simulink model "cccvlgorithmfinall"  (R2018b)
settings: Solver=VariableStepAuto  StartTime=0.0  StopTime=400  RelTol=1e-3
undefined symbols (not defined in the file): Ion, Lithium
libraries: powerlib x24, simulink x4, electricdrivelib x1, powerlib_meascontrol x1
settings Model: Creator=PARTO  LastModifiedBy=PARTO

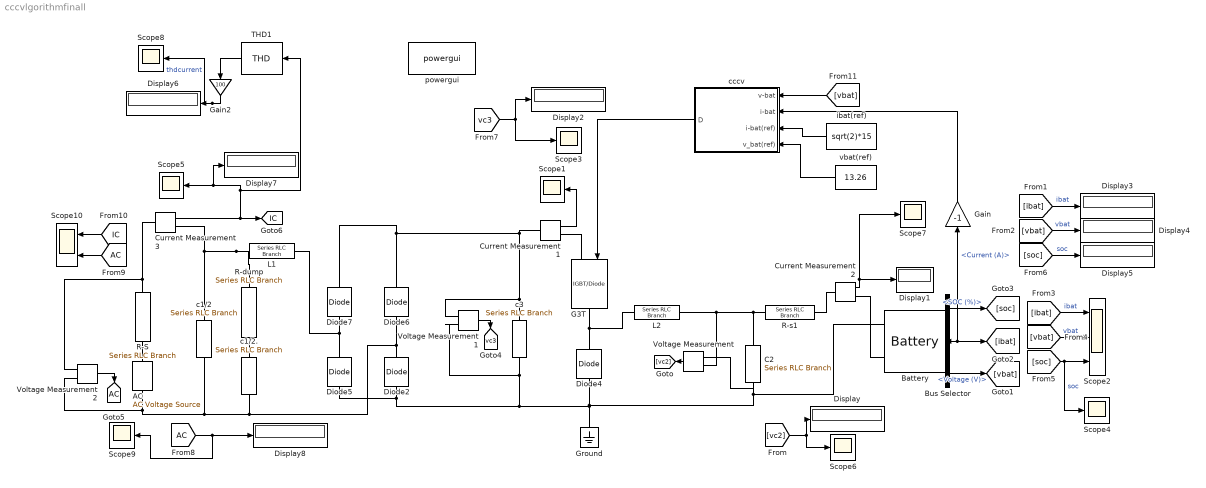
== system cccvlgorithmfinall ==
  AC : powerlib/Electrical Sources/AC Voltage Source  Amplitude=sqrt(2)*220  Phase=0  Frequency=50  SampleTime=0  Measurements=Voltage  BusType=PV  Pref=3.3e3  Qref=0  Qmin=-inf  Qmax=+inf
      settings: SourceProductName=Simscape Electrical
  Battery : electricdrivelib/Extra Sources/Battery  BatType=Lithium-Ion  ShowTempParam=off  ThermalPreset=no  ShowAgeParam=off  NomV=11.4  NomQ=5.4  SOC=19  Batt_Tr=30  PresetModel=on  MaxQ=5.4  MinV=8.55  FullV=13.2695  Dis_rate=2.3478  R=0.021111  Normal_OP=4.8835  expZone="[12.3164     0.265304]"  current=[6.5 13 32.5]  Units=Time  Tci=20  NomT=20  T2=-30  MaxQ2=4.8  FullV2=7.1  Normal_OP2=5.655  expZone2="[6.58           1]"  Rca=0.6  ti=2000  Dp=0  Neq0=0  Tsim=1e6  Ta1=25  Qeol=5.4*0.9  Reol=0.013333*1.2  Char_age=[2.3478, 3]  Dis_age=[2.3478, 10]  N1=1500  N2=10500  N3=1000  N4=1400  Ta2=45  N5=950
      settings: SourceProductName=Simscape Electrical
  Bus Selector : BusSelector  OutputSignals=SOC (%),Current (A),Voltage (V)
  C2 : powerlib/Elements/Series RLC Branch  LConnTagsString=__new0  RConnTagsString=__new0  BranchType=C  Resistance=1  Inductance=1e-3  SetiL0=off  InitialCurrent=0  Capacitance=700e-6  Setx0=off  InitialVoltage=0  Measurements=None
      settings: SourceProductName=Simscape Electrical
  Current Measurement1 : powerlib/Measurements/Current Measurement  PhasorSimulation=off  OutputType=Complex  PSBequivalent=0
      settings: SourceProductName=Simscape Electrical
  Current Measurement2 : powerlib/Measurements/Current Measurement  PhasorSimulation=off  OutputType=Complex  PSBequivalent=0
      settings: SourceProductName=Simscape Electrical
  Current Measurement3 : powerlib/Measurements/Current Measurement  PhasorSimulation=off  OutputType=Complex  PSBequivalent=0
      settings: SourceProductName=Simscape Electrical
  Diode{2,5..7} (4 alike) : powerlib/Power Electronics/Diode  Ron=0.000002  Lon=0.000002  Vf=0.8  IC=0  UseSnubber=0  Rs=0  Cs=0  Measurements=off
      settings: SourceProductName=Simscape Electrical
  Diode4 : powerlib/Power Electronics/Diode  Ron=0  Lon=0  Vf=0.8  IC=0  UseSnubber=0  Rs=0  Cs=0  Measurements=off
      settings: SourceProductName=Simscape Electrical
  Display{,1..8} (9 alike) : Display
  G3T : powerlib/Power Electronics/IGBT//Diode  Ron=1e-3  Rs=1e5  Cs=inf  Measurements=off
      settings: SourceProductName=Simscape Electrical
  Gain : Gain  Gain=-1
  Gain2 : Gain  Gain=100
  Ground : powerlib/Elements/Ground  LConnTagsString=a
      settings: SourceProductName=Simscape Electrical
  L1 : powerlib/Elements/Series RLC Branch  LConnTagsString=__new0  RConnTagsString=__new0  BranchType=L  Resistance=1  Inductance=5e-3  SetiL0=off  InitialCurrent=0  Capacitance=1e-6  Setx0=off  InitialVoltage=0  Measurements=None
      settings: SourceProductName=Simscape Electrical
  L2 : powerlib/Elements/Series RLC Branch  LConnTagsString=__new0  RConnTagsString=__new0  BranchType=L  Resistance=1  Inductance=1.5e-3  SetiL0=off  InitialCurrent=0  Capacitance=1e-6  Setx0=off  InitialVoltage=0  Measurements=None
      settings: SourceProductName=Simscape Electrical
  R-S : powerlib/Elements/Series RLC Branch  LConnTagsString=__new0  RConnTagsString=__new0  BranchType=R  Resistance=1e-6  Inductance=1e-3  SetiL0=off  InitialCurrent=0  Capacitance=1e-6  Setx0=off  InitialVoltage=0  Measurements=None
      settings: SourceProductName=Simscape Electrical
  "R-dump " : powerlib/Elements/Series RLC Branch  LConnTagsString=__new0  RConnTagsString=__new0  BranchType=R  Resistance=128  Inductance=1e-3  SetiL0=off  InitialCurrent=0  Capacitance=1e-6  Setx0=off  InitialVoltage=0  Measurements=None
      settings: SourceProductName=Simscape Electrical
  R-s1 : powerlib/Elements/Series RLC Branch  LConnTagsString=__new0  RConnTagsString=__new0  BranchType=R  Resistance=0.005  Inductance=1e-3  SetiL0=off  InitialCurrent=0  Capacitance=1e-6  Setx0=off  InitialVoltage=0  Measurements=None
      settings: SourceProductName=Simscape Electrical
  Scope{1,3..9} (8 alike) : Scope
  Scope10 : Scope  NumInputPorts=2
  Scope2 : Scope  NumInputPorts=3
  THD1 : powerlib_meascontrol/Measurements/THD  Freq=50  Ts=0
      settings: SourceProductName=Simscape Electrical
  Voltage Measurement : powerlib/Measurements/Voltage Measurement  PhasorSimulation=off  OutputType=Complex  PSBequivalent=0
      settings: SourceProductName=Simscape Electrical
  Voltage Measurement1 : powerlib/Measurements/Voltage Measurement  PhasorSimulation=off  OutputType=Complex  PSBequivalent=0
      settings: SourceProductName=Simscape Electrical
  Voltage Measurement2 : powerlib/Measurements/Voltage Measurement  PhasorSimulation=off  OutputType=Complex  PSBequivalent=0
      settings: SourceProductName=Simscape Electrical
  c1/2 : powerlib/Elements/Series RLC Branch  LConnTagsString=__new0  RConnTagsString=__new0  BranchType=C  Resistance=1  Inductance=1e-3  SetiL0=off  InitialCurrent=0  Capacitance=250e-6  Setx0=off  InitialVoltage=0  Measurements=None
      settings: SourceProductName=Simscape Electrical
  c1/2. : powerlib/Elements/Series RLC Branch  LConnTagsString=__new0  RConnTagsString=__new0  BranchType=C  Resistance=1  Inductance=1e-3  SetiL0=off  InitialCurrent=0  Capacitance=250e-6  Setx0=off  InitialVoltage=0  Measurements=None
      settings: SourceProductName=Simscape Electrical
  c3 : powerlib/Elements/Series RLC Branch  LConnTagsString=__new0  RConnTagsString=__new0  BranchType=C  Resistance=1  Inductance=1e-3  SetiL0=off  InitialCurrent=0  Capacitance=1000e-6  Setx0=off  InitialVoltage=0  Measurements=None
      settings: SourceProductName=Simscape Electrical
  cccv : Subsystem
  ibat(ref) : Constant  Value=sqrt(2)*15
  powergui : powerlib/powergui  Priority=1  SimulationMode=Continuous  SampleTime=50e-6  frequency=60  Iterations=50  frequencyindice=0  Pbase=100e6  ErrMax=1e-4  UnitsV=kV  UnitsW=MW  buscounter=0  FunctionMessages=off  echomessages=off  EnableUseOfTLC=off  CurrentSourceSwitches=off  DisableSnubberDevices=off  DisableRonSwitches=off  DisableVfSwitches=off  DisplayEquations=off  SolverType=Tustin/Backward Euler (TBE)  Interpol=off  ExternalGateDelay=off  methode=off  Ts=100  x0status=blocks  SPID=on  SwTol=0  HookPort=off  RestoreLinks=warning  ResistiveCurrentMeasurement=off  Frange=[0:2:500]  Ylog=off  Xlog=on  ShowGrid=off  save=off  variable=ZData  structure=0  ZoomFFT=off  StartTime=0.0  cycles=1  DisplayStyle=1  fundamental=60  FreqAxis=off  MaxFrequency=1000  frequencyindicesteady=1  RmsSteady=1  display=off
  vbat(ref) : Constant  Value=13.26
  tag scope: AC=global, IC=global, vc3=global
  wires:
  Current Measurement2/1 -> Scope7/1, Display1/1
  Bus Selector/2 -> [ibat], Gain/1  "<Current (A)>"
  Battery/1 -> Bus Selector/1
  Current Measurement1/1 -> Scope1/1
  Voltage Measurement/1 -> [vc2]
  [vc2] -> Scope6/1, Display/1
  [ibat] -> Scope2/1  "ibat"
  Bus Selector/1 -> [soc]  "<SOC (%)>"
  [soc] -> Scope4/1, Scope2/3  "soc"
  [vbat] -> Scope2/2  "vbat"
  Bus Selector/3 -> [vbat]  "<Voltage (V)>"
  [ibat] -> Display3/1  "ibat"
  [vbat] -> Display4/1  "vbat"
  [soc] -> Display5/1  "soc"
  THD1/1 -> Gain2/1
  Gain2/1 -> Scope8/1, Display6/1  "thdcurrent"
  Current Measurement3/1 -> [IC], THD1/1, Display7/1, Scope5/1
  Voltage Measurement1/1 -> [vc3]
  [vc3] -> Display2/1, Scope3/1
  Voltage Measurement2/1 -> [AC]
  [AC] -> Scope9/1, Display8/1
  [IC] -> Scope10/1
  [AC] -> Scope10/2
  Gain/1 -> cccv/2(i-bat)
  [vbat] -> cccv/1(v-bat)
  cccv/1(D) -> G3T/1
  ibat(ref)/1 -> cccv/3(i-bat(ref))
  vbat(ref)/1 -> cccv/4(v_bat(ref))
  connections:
  Battery/LConn2 -- Ground/LConn1 -- c3/RConn1 -- Voltage Measurement1/LConn2 -- Diode2/LConn1 -- Diode5/LConn1 -- Diode4/LConn1 -- Voltage Measurement/LConn2 -- C2/RConn1
  G3T/RConn1 -- Diode4/RConn1 -- L2/LConn1
  c3/LConn1 -- Voltage Measurement1/LConn1 -- Diode6/RConn1 -- Diode7/RConn1 -- Current Measurement1/LConn1
  L1/LConn1 -- "R-dump "/LConn1 -- c1/2/LConn1 -- Current Measurement3/RConn1
  Diode6/LConn1 -- Diode2/RConn1 -- c1/2./RConn1 -- Voltage Measurement2/LConn2 -- AC/LConn1 -- c1/2/RConn1
  Diode5/RConn1 -- L1/RConn1 -- Diode7/LConn1
  R-s1/LConn1 -- L2/RConn1 -- Voltage Measurement/LConn1 -- C2/LConn1
  R-s1/RConn1 -- Current Measurement2/LConn1
  Current Measurement1/RConn1 -- G3T/LConn1
  Current Measurement2/RConn1 -- Battery/LConn1
  "R-dump "/RConn1 -- c1/2./LConn1
  Current Measurement3/LConn1 -- Voltage Measurement2/LConn1 -- R-S/RConn1
  AC/RConn1 -- R-S/LConn1

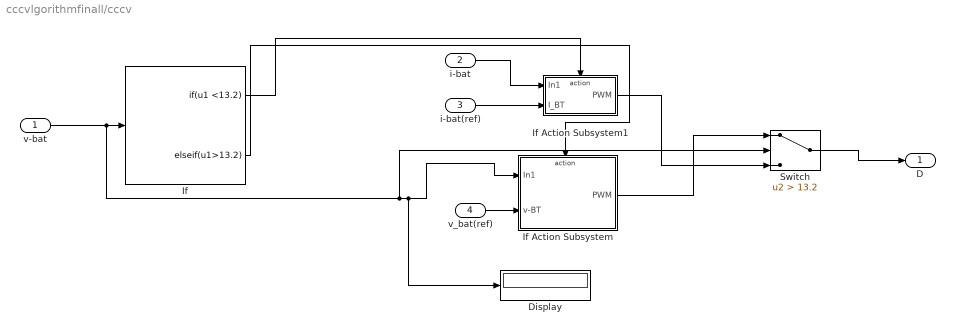
== system cccvlgorithmfinall/cccv ==
  v-bat : Inport
  i-bat : Inport  Port=2
  i-bat(ref) : Inport  Port=3
  v_bat(ref) : Inport  Port=4
  Display : Display
  If : If  IfExpression=u1 <13.2  ElseIfExpressions=u1>13.2  ShowElse=off
  If Action Subsystem : Subsystem  TreatAsAtomicUnit=on
  If Action Subsystem1 : Subsystem  TreatAsAtomicUnit=on
  Switch : Switch  Criteria=u2 > Threshold  Threshold=13.2
  D : Outport
  wires:
  If/1 -> If Action Subsystem1/Action
  i-bat/1 -> If Action Subsystem1/1(In1)
  If/2 -> If Action Subsystem/Action
  i-bat(ref)/1 -> If Action Subsystem1/2(I_BT)
  v_bat(ref)/1 -> If Action Subsystem/2(v-BT)
  v-bat/1 -> Switch/2, Display/1, If Action Subsystem/1(In1), If/1
  If Action Subsystem/1(PWM) -> Switch/1
  If Action Subsystem1/1(PWM) -> Switch/3
  Switch/1 -> D/1

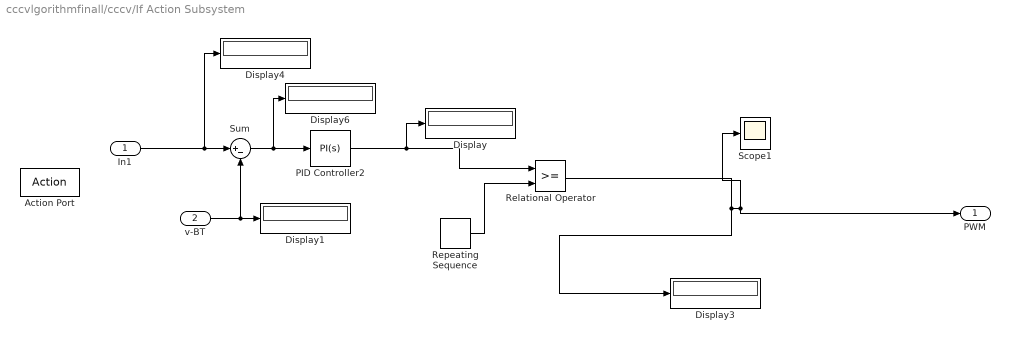
== system cccvlgorithmfinall/cccv/If Action Subsystem ==
  In1 : Inport
  v-BT : Inport  Port=2
  Action Port : ActionPort  ActionType=elseif
  Display{,1,3..4,6} (5 alike) : Display
  PID Controller2 : simulink/Continuous/PID Controller  Controller=PI  Form=Parallel  TimeDomain=Continuous-time  SampleTime=-1  IntegratorMethod=Forward Euler  FilterMethod=Forward Euler  ControllerParametersSource=internal  P=100  I=1  D=0  UseFilter=on  N=100  TunerSelectOption=Transfer Function Based (PID Tuner App)  InitialConditionSource=internal  InitialConditionForIntegrator=0  InitialConditionForFilter=0  DifferentiatorICPrevScaledInput=0  ExternalReset=none  TrackingMode=off  Kt=1  LimitOutput=off  UpperSaturationLimit=inf  LowerSaturationLimit=-inf  LinearizeAsGain=on  AntiWindupMode=none  Kb=1  POutMin=[]  POutMax=[]  IOutMin=[]  IOutMax=[]  DOutMin=[]  DOutMax=[]  NOutMin=[]  NOutMax=[]  SumOutMin=[]  SumOutMax=[]  SaturationOutMin=[]  SaturationOutMax=[]  PParamMin=[]  PParamMax=[]  IParamMin=[]  IParamMax=[]  DParamMin=[]  DParamMax=[]  NParamMin=[]  NParamMax=[]  KbParamMin=[]  KbParamMax=[]  KtParamMin=[]  KtParamMax=[]  KbOutMin=[]  KbOutMax=[]  KtOutMin=[]  KtOutMax=[]  IntegratorOutMin=[]  IntegratorOutMax=[]  FilterOutMin=[]  FilterOutMax=[]  SumI1OutMin=[]  SumI1OutMax=[]  SumI2OutMin=[]  SumI2OutMax=[]  SumI3OutMin=[]  SumI3OutMax=[]  SumI4OutMin=[]  SumI4OutMax=[]  SumDOutMin=[]  SumDOutMax=[]  DifferentiatorOutMin=[]  DifferentiatorOutMax=[]  FilterDiffOutCoefMin=[]  FilterDiffOutCoefMax=[]  ReciprocalOutMin=[]  ReciprocalOutMax=[]  SumDenOutMin=[]  SumDenOutMax=[]  SumNumOutMin=[]  SumNumOutMax=[]  DivideOutMin=[]  DivideOutMax=[]  IntegratorContinuousStateAttributes=''  IntegratorStateMustResolveToSignalObject=off  IntegratorRTWStateStorageClass=Auto  FilterContinuousStateAttributes=''  FilterStateMustResolveToSignalObject=off  FilterRTWStateStorageClass=Auto  ParallelPVariant=InternalParameters  IdealPVariant=Disabled  IVariant=InternalParameters  DVariant=Disabled  IntegratorVariant=Continuous  SatVariant=Disabled  AWVariant=Passthrough  PCopyVariant=Disabled  TRVariant=Disabled  FdbkBlocksVariant=Forward  IdealPFdbkVariant=Disabled  SatFdbkVariant=Disabled  DerivativeFilterVariant=Disabled  NVariant=Disabled  NCopyVariant=Disabled_SignalSpec  FilterICVariant=Disabled  IntegratorICVariant=InternalICs  ExternalResetVariant=Disabled  TRSumVariant=Passthrough  SumFdbkVariant=Disabled  SumVariant=Sum_PI
  Relational Operator : RelationalOperator  OutDataTypeStr=boolean  RndMeth=Simplest
  Repeating Sequence : simulink/Sources/Repeating Sequence  rep_seq_t=[0 1/40e3]  rep_seq_y=[0 1]
  Scope1 : Scope
  Sum : Sum  Inputs=|+-
  PWM : Outport
  wires:
  Repeating Sequence/1 -> Relational Operator/2
  PID Controller2/1 -> Display/1, Relational Operator/1
  Sum/1 -> PID Controller2/1, Display6/1
  v-BT/1 -> Sum/2, Display1/1
  In1/1 -> Sum/1, Display4/1
  Relational Operator/1 -> Display3/1, PWM/1, Scope1/1

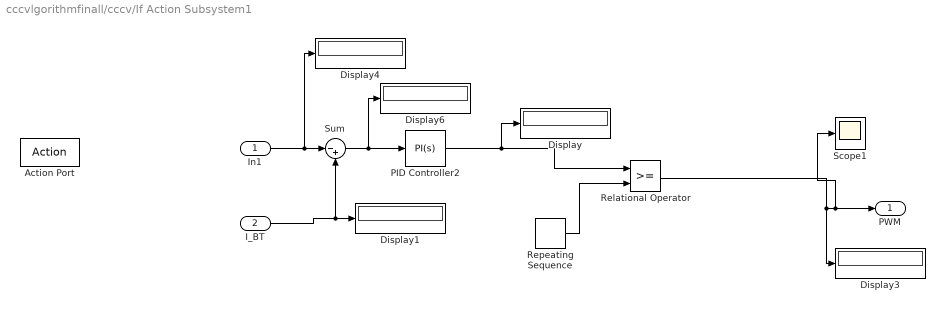
== system cccvlgorithmfinall/cccv/If Action Subsystem1 ==
  In1 : Inport
  I_BT : Inport  Port=2
  Action Port : ActionPort  ActionType=then
  Display{,1,3..4,6} (5 alike) : Display
  PID Controller2 : simulink/Continuous/PID Controller  Controller=PI  Form=Parallel  TimeDomain=Continuous-time  SampleTime=-1  IntegratorMethod=Forward Euler  FilterMethod=Forward Euler  ControllerParametersSource=internal  P=1  I=0.001  D=0  UseFilter=on  N=100  TunerSelectOption=Transfer Function Based (PID Tuner App)  InitialConditionSource=internal  InitialConditionForIntegrator=0  InitialConditionForFilter=0  DifferentiatorICPrevScaledInput=0  ExternalReset=none  TrackingMode=off  Kt=1  LimitOutput=off  UpperSaturationLimit=inf  LowerSaturationLimit=-inf  LinearizeAsGain=on  AntiWindupMode=none  Kb=1  POutMin=[]  POutMax=[]  IOutMin=[]  IOutMax=[]  DOutMin=[]  DOutMax=[]  NOutMin=[]  NOutMax=[]  SumOutMin=[]  SumOutMax=[]  SaturationOutMin=[]  SaturationOutMax=[]  PParamMin=[]  PParamMax=[]  IParamMin=[]  IParamMax=[]  DParamMin=[]  DParamMax=[]  NParamMin=[]  NParamMax=[]  KbParamMin=[]  KbParamMax=[]  KtParamMin=[]  KtParamMax=[]  KbOutMin=[]  KbOutMax=[]  KtOutMin=[]  KtOutMax=[]  IntegratorOutMin=[]  IntegratorOutMax=[]  FilterOutMin=[]  FilterOutMax=[]  SumI1OutMin=[]  SumI1OutMax=[]  SumI2OutMin=[]  SumI2OutMax=[]  SumI3OutMin=[]  SumI3OutMax=[]  SumI4OutMin=[]  SumI4OutMax=[]  SumDOutMin=[]  SumDOutMax=[]  DifferentiatorOutMin=[]  DifferentiatorOutMax=[]  FilterDiffOutCoefMin=[]  FilterDiffOutCoefMax=[]  ReciprocalOutMin=[]  ReciprocalOutMax=[]  SumDenOutMin=[]  SumDenOutMax=[]  SumNumOutMin=[]  SumNumOutMax=[]  DivideOutMin=[]  DivideOutMax=[]  IntegratorContinuousStateAttributes=''  IntegratorStateMustResolveToSignalObject=off  IntegratorRTWStateStorageClass=Auto  FilterContinuousStateAttributes=''  FilterStateMustResolveToSignalObject=off  FilterRTWStateStorageClass=Auto  ParallelPVariant=InternalParameters  IdealPVariant=Disabled  IVariant=InternalParameters  DVariant=Disabled  IntegratorVariant=Continuous  SatVariant=Disabled  AWVariant=Passthrough  PCopyVariant=Disabled  TRVariant=Disabled  FdbkBlocksVariant=Forward  IdealPFdbkVariant=Disabled  SatFdbkVariant=Disabled  DerivativeFilterVariant=Disabled  NVariant=Disabled  NCopyVariant=Disabled_SignalSpec  FilterICVariant=Disabled  IntegratorICVariant=InternalICs  ExternalResetVariant=Disabled  TRSumVariant=Passthrough  SumFdbkVariant=Disabled  SumVariant=Sum_PI
  Relational Operator : RelationalOperator  OutDataTypeStr=boolean  RndMeth=Simplest
  Repeating Sequence : simulink/Sources/Repeating Sequence  rep_seq_t=[0 1/40e3]  rep_seq_y=[0 1]
  Scope1 : Scope
  Sum : Sum  Inputs=|-+
  PWM : Outport
  wires:
  Relational Operator/1 -> Display3/1, Scope1/1, PWM/1
  PID Controller2/1 -> Display/1, Relational Operator/1
  Sum/1 -> PID Controller2/1, Display6/1
  Repeating Sequence/1 -> Relational Operator/2
  I_BT/1 -> Sum/2, Display1/1
  In1/1 -> Display4/1, Sum/1
